simulink model "Moteur_Causal"  (R2016b)
settings: Solver=VariableStepAuto  StartTime=0.0  StopTime=.1  RelTol=1e-3
undefined symbols (not defined in the file): J, Ke, L, R
settings Model: Creator=Xavier  LastModifiedBy=Xavier

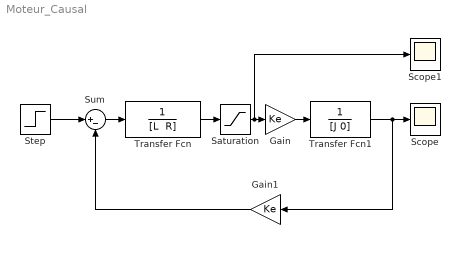
== system Moteur_Causal ==
  Gain : Gain  Gain=Ke
  Gain1 : Gain  Gain=Ke
  Saturation : Saturate  UpperLimit=8  LowerLimit=-8
  Scope : Scope
  Scope1 : Scope
  Step : Step  Time=0  After=48  SampleTime=0
  Sum : Sum  Inputs=|+-
  Transfer Fcn : TransferFcn  Denominator="[L  R]"
  Transfer Fcn1 : TransferFcn  Denominator=[J 0]
  wires:
  Sum/1 -> Transfer Fcn/1
  Gain/1 -> Transfer Fcn1/1
  Transfer Fcn1/1 -> Gain1/1, Scope/1
  Gain1/1 -> Sum/2
  Step/1 -> Sum/1
  Transfer Fcn/1 -> Saturation/1
  Saturation/1 -> Scope1/1, Gain/1
